simulink model "Kundur_BESS_STA_Nov14_2021a_v2_2021a"  (R2023a)
settings: Solver=VariableStepAuto  StartTime=0.0  StopTime=3  FixedStep=Ts  MaxStep=1e-5  MinStep=1e-20  RelTol=1e-3  EnableMultiTasking=on
PreLoadFcn:
  | Ts=50e-6;
PostLoadFcn:
  | Ts=50e-6;
InitFcn:
  | Ts=50e-6;
values from neighbouring files (symbols this model uses):
  current_K_den = [1 -1.95396088137 0.953960881373]    [param_cntrl_v2.mat]
  current_K_num = [292.549944556 -582.765243791 290.215658722]    [param_cntrl_v2.mat]
  flt_den = [1 -1.99914493247 0.999500180349]    [param_cntrl_v2.mat]
  flt_num = [0.000249925443627 3.12366678454e-08 -0.000249894206959]    [param_cntrl_v2.mat]
  flt_rocof_den = [1 -3.94812243331 5.84544117496 -3.84650440967 0.949185710471]    [param_cntrl_v2.mat]
  flt_rocof_num = [2.65341753303e-09 1.06136701321e-08 1.59205051982e-08 1.06136701321e-08 2.65341753303e-09]    [param_cntrl_v2.mat]
  pll_K_den = [1 -1.95396088137 0.953960881373]    [param_cntrl_v2.mat]
  pll_K_num = [1047.77474974 -2078.89023245 1031.12061217]    [param_cntrl_v2.mat]
  sampling_k = 5e-05    [param_cntrl_v2.mat]
undefined symbols (not defined in the file or in its folder): Ad2, Ad4, Bd2, Bd4, Cd2, Cd4, D1, Delta, flt_rocof_a_den, flt_rocof_a_num, flt_rocof_b_den, flt_rocof_b_num, Gd2, Gd4, Kd2, Kd4, L, R
libraries: spsThreePhaseVIMeasurementLib x15, spsLoadFlowBusLib x12, spsSeriesRLCBranchLib x11, spsThreePhaseSeriesRLCLoadLib x11, spsThreePhaseTransformerTwoWindingsLib x8, spsThreePhaseSeriesRLCBranchLib x8, spsabctoAlphaBetaZeroLib x8, spsGenericPowerSystemStabilizerLib x8, spsPowerPositiveSequenceLib x7, spsThreePhaseParallelRLCLoadLib x6, spsPLL3phLib x6, spsGroundLib x6
(part 3 of 4)

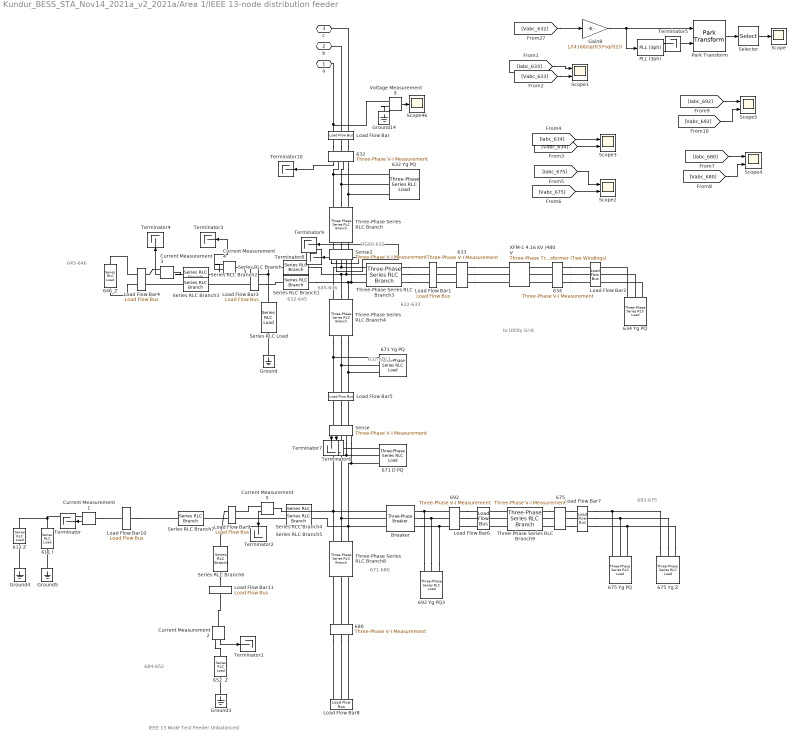
== system Kundur_BESS_STA_Nov14_2021a_v2_2021a/Area 1/IEEE 13-node distribution feeder ==
  note: 632-633
  note: 645-646
  note: 684-652
  note: 692-675
  note: 671-680
  note: 632-nDL1
  note: IEEE 13 Node Test Feeder Unbalanced
  note: 632-645
  note: RG60-632
  note: to Utility Grid
  note: 645-646
  " 634 Yg PQ " : spsThreePhaseSeriesRLCLoadLib/Three-Phase Series RLC Load  LConnTagsString=A|B|C  Configuration=Y (grounded)  NominalVoltage=120e3  Vabc=[ 1 1 1]*277.128  Vabcp=[1e3 1e3 1e3]  NominalFrequency=60  UnbalancedPower=on  ActivePower=1e+006  InductivePower=0  CapacitivePower=0  Pabc=[160 120 120]*1e3  QLabc=[110 90 90]*1e3  QCabc=[0 0 0]  Pabcp=[10e3 9e3 11e3]  QLabcp=[100 90 110]  QCabcp=[100 90 110]  Measurements=None  LoadType=constant PQ
      settings: AttributesFormatString=|
      | P= %<Pabc> W
      | Ql=%<QLabc> var
      | Qc=%<QCabc> var
  611 I : spsSeriesRLCLoadLib/Series RLC Load  LConnTagsString=a  RConnTagsString=__new0  NominalVoltage=0.986941*2401.78  NominalFrequency=60  ActivePower=50e3  InductivePower=80e3  CapacitivePower=0  Setx0=off  InitialVoltage=0  SetiL0=off  InitialCurrent=0  Measurements=None  LoadType=constant I
      settings: AttributesFormatString=|
      | P=%<ActivePower> W
      | Ql=%<InductivePower> var
      | Qc=%<CapacitivePower> var
  611 Z : spsSeriesRLCLoadLib/Series RLC Load  LConnTagsString=a  RConnTagsString=__new0  NominalVoltage=4160/sqrt(3)  NominalFrequency=60  ActivePower=0  InductivePower=0  CapacitivePower=100e3  Setx0=off  InitialVoltage=0  SetiL0=off  InitialCurrent=0  Measurements=None  LoadType=constant Z
      settings: AttributesFormatString=|
      | P=%<ActivePower> W
      | Ql=%<InductivePower> var
      | Qc=%<CapacitivePower> var
  632 : spsThreePhaseVIMeasurementLib/Three-Phase V-I Measurement  VoltageMeasurement=phase-to-ground  SetLabelV=on  LabelV=Vabc_632  Vpu=off  VpuLL=off  CurrentMeasurement=yes  SetLabelI=off  LabelI=Iabc_632  Ipu=off  Pbase=100e6  Vbase=4160  OutputType=Complex  PhasorSimulation=off  PSBequivalent=0
  632 Yg PQ : spsThreePhaseSeriesRLCLoadLib/Three-Phase Series RLC Load  LConnTagsString=A|B|C  Configuration=Y (grounded)  NominalVoltage=120e3  Vabc=[ 1.021 1.042 1.0174]*2401.78  Vabcp=[1e3 1e3 1e3]  NominalFrequency=60  UnbalancedPower=on  ActivePower=1e+006  InductivePower=0  CapacitivePower=0  Pabc="[17 66  117]*1e3/2"  QLabc="[10 38  68]*1e3/2"  QCabc=[0 0 0]  Pabcp=[10e3 9e3 11e3]  QLabcp=[100 90 110]  QCabcp=[100 90 110]  Measurements=None  LoadType=constant PQ
      settings: AttributesFormatString=|
      | P= %<Pabc> W
      | Ql=%<QLabc> var
      | Qc=%<QCabc> var
  633 : spsThreePhaseVIMeasurementLib/Three-Phase V-I Measurement  VoltageMeasurement=phase-to-ground  SetLabelV=on  LabelV=Vabc_633  Vpu=off  VpuLL=off  CurrentMeasurement=yes  SetLabelI=on  LabelI=Iabc_633  Ipu=off  Pbase=100e6  Vbase=4160  OutputType=Complex  PhasorSimulation=off  PSBequivalent=0
  634 : spsThreePhaseVIMeasurementLib/Three-Phase V-I Measurement  VoltageMeasurement=phase-to-ground  SetLabelV=on  LabelV=Vabc_634  Vpu=off  VpuLL=off  CurrentMeasurement=yes  SetLabelI=on  LabelI=Iabc_634  Ipu=off  Pbase=100e6  Vbase=4160  OutputType=Complex  PhasorSimulation=off  PSBequivalent=0
  646_Z : spsSeriesRLCLoadLib/Series RLC Load  LConnTagsString=a  RConnTagsString=__new0  NominalVoltage=4160  NominalFrequency=60  ActivePower=30e3  InductivePower=132e3  CapacitivePower=0  Setx0=off  InitialVoltage=0  SetiL0=off  InitialCurrent=0  Measurements=None  LoadType=constant Z
      settings: AttributesFormatString=|
      | P=%<ActivePower> W
      | Ql=%<InductivePower> var
      | Qc=%<CapacitivePower> var
  "652  Z " : spsSeriesRLCLoadLib/Series RLC Load  LConnTagsString=a  RConnTagsString=__new0  NominalVoltage=4160/sqrt(3)  NominalFrequency=60  ActivePower=128e3*0.1  InductivePower=86e3  CapacitivePower=0  Setx0=off  InitialVoltage=0  SetiL0=off  InitialCurrent=0  Measurements=None  LoadType=constant Z
      settings: AttributesFormatString=|
      | P=%<ActivePower> W
      | Ql=%<InductivePower> var
      | Qc=%<CapacitivePower> var
  671 D PQ : spsThreePhaseSeriesRLCLoadLib/Three-Phase Series RLC Load  LConnTagsString=A|B|C  Configuration=Delta  NominalVoltage=120e3  Vabc="[1  1  1]*120e3/sqrt(3)"  Vabcp=[ 1.73773 1.77224 1.71484]*2401.78  NominalFrequency=60  UnbalancedPower=on  ActivePower=1e+006  InductivePower=0  CapacitivePower=0  Pabc="[17 66  117]*1e3/2"  QLabc="[10 38  68]*1e3/2"  QCabc=[0 0 0]  Pabcp=[385 385 385 ]*1e3  QLabcp=[220 220 220]*1e3  QCabcp="[0  0  0]"  Measurements=None  LoadType=constant PQ
      settings: AttributesFormatString=|
      | P= %<Pabcp> W
      | Ql=%<QLabcp> var
      | Qc=%<QCabcp> var
  671 Yg PQ : spsThreePhaseSeriesRLCLoadLib/Three-Phase Series RLC Load  LConnTagsString=A|B|C  Configuration=Y (grounded)  NominalVoltage=120e3  Vabc=[ 0.987076 1.0519 0.978043]*2401.78  Vabcp=[1e3 1e3 1e3]  NominalFrequency=60  UnbalancedPower=on  ActivePower=1e+006  InductivePower=0  CapacitivePower=0  Pabc="[17 66  117]*1e3/2"  QLabc="[10 38  68]*1e3/2"  QCabc=[0 0 0]  Pabcp=[10e3 9e3 11e3]  QLabcp=[100 90 110]  QCabcp=[100 90 110]  Measurements=None  LoadType=constant PQ
      settings: AttributesFormatString=|
      | P= %<Pabc> W
      | Ql=%<QLabc> var
      | Qc=%<QCabc> var
  675 : spsThreePhaseVIMeasurementLib/Three-Phase V-I Measurement  VoltageMeasurement=phase-to-ground  SetLabelV=on  LabelV=Vabc_675  Vpu=off  VpuLL=off  CurrentMeasurement=yes  SetLabelI=on  LabelI=Iabc_675  Ipu=off  Pbase=100e6  Vbase=4160  OutputType=Complex  PhasorSimulation=off  PSBequivalent=0
  675 Yg PQ : spsThreePhaseSeriesRLCLoadLib/Three-Phase Series RLC Load  LConnTagsString=A|B|C  Configuration=Y (grounded)  NominalVoltage=120e3  Vabc=[ 0.98063 1.05431 0.975983]*2401.78  Vabcp=[1e3 1e3 1e3]  NominalFrequency=60  UnbalancedPower=on  ActivePower=1e+006  InductivePower=0  CapacitivePower=0  Pabc="[485  68  290]*1e3"  QLabc="[190  60  212]*1e3"  QCabc=[0 0 0]  Pabcp=[10e3 9e3 11e3]  QLabcp=[100 90 110]  QCabcp=[100 90 110]  Measurements=None  LoadType=constant PQ
      settings: AttributesFormatString=|
      | P= %<Pabc> W
      | Ql=%<QLabc> var
      | Qc=%<QCabc> var
  675 Yg Z : spsThreePhaseSeriesRLCLoadLib/Three-Phase Series RLC Load  LConnTagsString=A|B|C  Configuration=Y (grounded)  NominalVoltage=120e3  Vabc=[ 1 1 1]*2401.78  Vabcp=[1e3 1e3 1e3]  NominalFrequency=60  UnbalancedPower=on  ActivePower=1e+006  InductivePower=0  CapacitivePower=0  Pabc=[0 0 0]  QLabc=[0 0 0]  QCabc=[200 200 200]*1e3  Pabcp=[10e3 9e3 11e3]  QLabcp=[100 90 110]  QCabcp=[100 90 110]  Measurements=None  LoadType=constant Z
      settings: AttributesFormatString=|
      | P= %<Pabc> W
      | Ql=%<QLabc> var
      | Qc=%<QCabc> var
  680 : spsThreePhaseVIMeasurementLib/Three-Phase V-I Measurement  VoltageMeasurement=phase-to-ground  SetLabelV=on  LabelV=Vabc_680  Vpu=off  VpuLL=off  CurrentMeasurement=yes  SetLabelI=on  LabelI=Iabc_680  Ipu=off  Pbase=100e6  Vbase=4160  OutputType=Complex  PhasorSimulation=off  PSBequivalent=0
  692 : spsThreePhaseVIMeasurementLib/Three-Phase V-I Measurement  VoltageMeasurement=phase-to-ground  SetLabelV=on  LabelV=Vabc_692  Vpu=off  VpuLL=off  CurrentMeasurement=yes  SetLabelI=on  LabelI=Iabc_692  Ipu=off  Pbase=100e6  Vbase=4160  OutputType=Complex  PhasorSimulation=off  PSBequivalent=0
  692 Yg PQ3 : spsThreePhaseSeriesRLCLoadLib/Three-Phase Series RLC Load  LConnTagsString=A|B|C  Configuration=Y (grounded)  NominalVoltage=120e3  Vabc=[ 1.73488 1.75203 1.72341]*2401.78  Vabcp=[1e3 1e3 1e3]  NominalFrequency=60  UnbalancedPower=on  ActivePower=1e+006  InductivePower=0  CapacitivePower=0  Pabc=[1e-6 1e-6 170 ]*1e3  QLabc=[3000 3000 3000]*1e3  QCabc=[0 0 0]  Pabcp=[10e3 9e3 11e3]  QLabcp=[100 90 110]  QCabcp=[100 90 110]  Measurements=None  LoadType=constant PQ
      settings: AttributesFormatString=|
      | P= %<Pabc> W
      | Ql=%<QLabc> var
      | Qc=%<QCabc> var
  Breaker : spsThreePhaseBreakerLib/Three-Phase Breaker  InitialState=closed  SwitchA=on  SwitchB=on  SwitchC=on  SwitchTimes=[0]  External=off  BreakerResistance=0.001  SnubberResistance=1e3  SnubberCapacitance=1e-4  Measurements=None
  Current Measurement{1..5} (5 alike) : spsCurrentMeasurementLib/Current Measurement  PhasorSimulation=off  OutputType=Complex  PSBequivalent=0
  Gain8 : Gain  Gain=1/(4160/sqrt(3)*sqrt(2))
  Ground{,3..5,14} (5 alike) : spsGroundLib/Ground  LConnTagsString=a
  Load Flow Bar : spsLoadFlowBusLib/Load Flow Bus  LConnTagsString=a|b|c  RConnTagsString=a|b|c  Phases=ABC  Connectors=on both sides  ID=632  Vbase=2401.78  Vref="[ 1  1  1]"  Vangle="[ 0  -120  120]"  VLF=1.021  VLFb=1.042  VLFc=1.017  angleLF=-2.49  angleLFb=-121.7  angleLFc=117.8
      settings: AttributesFormatString=%<ID>
  Load Flow Bar1 : spsLoadFlowBusLib/Load Flow Bus  LConnTagsString=a|b|c  RConnTagsString=a|b|c  Phases=ABC  Connectors=on both sides  ID=633  Vbase=2401.78  Vref=[1.0 1.0 1.0]  Vangle=[0 -120 120]  VLF=0.9671  VLFb=0.9801  VLFc=0.9575  angleLF=-5.793  angleLFb=-125.9  angleLFc=113.9
      settings: AttributesFormatString=%<ID>
  Load Flow Bar10 : spsLoadFlowBusLib/Load Flow Bus  LConnTagsString=a  RConnTagsString=a  Phases=C  Connectors=on both sides  ID=611  Vbase=2401.78  Vref=[1.0 1.0 1.0]  Vangle=[0 -120 120]  VLF=NaN  VLFb=NaN  VLFc=0.9623  angleLF=NaN  angleLFb=NaN  angleLFc=112.9
      settings: AttributesFormatString=%<ID>
  Load Flow Bar11 : spsLoadFlowBusLib/Load Flow Bus  LConnTagsString=a  RConnTagsString=a  Phases=A  Connectors=on both sides  ID=652  Vbase=2401.78  Vref=[1.0 1.0 1.0]  Vangle=[0 -120 120]  VLF=0.969  VLFb=NaN  VLFc=NaN  angleLF=-6.548  angleLFb=NaN  angleLFc=NaN
      settings: AttributesFormatString=%<ID>
  Load Flow Bar2 : spsLoadFlowBusLib/Load Flow Bus  LConnTagsString=a|b|c  RConnTagsString=a|b|c  Phases=ABC  Connectors=on both sides  ID=634  Vbase=480/sqrt(3)  Vref="[1  1  1 ]"  Vangle=[0 -120 120]  VLF=0.9473  VLFb=0.9605  VLFc=0.9374  angleLF=-6.323  angleLFb=-126.4  angleLFc=113.4
      settings: AttributesFormatString=%<ID>
  Load Flow Bar3 : spsLoadFlowBusLib/Load Flow Bus  LConnTagsString=a|b  RConnTagsString=a|b  Phases=BC  Connectors=on both sides  ID=645  Vbase=2401.78  Vref=[1 1 1]  Vangle=[0 -120 120]  VLF=NaN  VLFb=0.982  VLFc=0.9645  angleLF=NaN  angleLFb=-126.4  angleLFc=113.8
      settings: AttributesFormatString=%<ID>
  Load Flow Bar4 : spsLoadFlowBusLib/Load Flow Bus  LConnTagsString=a|b  RConnTagsString=a|b  Phases=BC  Connectors=on both sides  ID=646  Vbase=2401.78  Vref=[1 1 1]  Vangle=[0 -120 120]  VLF=NaN  VLFb=0.9803  VLFc=0.9619  angleLF=NaN  angleLFb=-126.5  angleLFc=113.8
      settings: AttributesFormatString=%<ID>
  Load Flow Bar5 : spsLoadFlowBusLib/Load Flow Bus  LConnTagsString=a|b|c  RConnTagsString=a|b|c  Phases=ABC  Connectors=on both sides  ID=671  Vbase=2401.78  Vref=[1.0 1.0 1.0]  Vangle=[0 -120 120]  VLF=0.9734  VLFb=0.988  VLFc=0.9653  angleLF=-6.515  angleLFb=-126.5  angleLFc=113.1
      settings: AttributesFormatString=%<ID>
  Load Flow Bar6 : spsLoadFlowBusLib/Load Flow Bus  LConnTagsString=a|b|c  RConnTagsString=a|b|c  Phases=ABC  Connectors=on both sides  ID=692  Vbase=2401.78  Vref=[1 1 1]  Vangle=[0 -120 120]  VLF=0.9734  VLFb=0.988  VLFc=0.9653  angleLF=-6.515  angleLFb=-126.5  angleLFc=113.1
      settings: AttributesFormatString=%<ID>
  Load Flow Bar7 : spsLoadFlowBusLib/Load Flow Bus  LConnTagsString=a|b|c  RConnTagsString=a|b|c  Phases=ABC  Connectors=on both sides  ID=675  Vbase=2401.78  Vref=[1 1 1]  Vangle=[0 -120 120]  VLF=0.9761  VLFb=0.9908  VLFc=0.9679  angleLF=-6.673  angleLFb=-126.7  angleLFc=113
      settings: AttributesFormatString=%<ID>
  Load Flow Bar8 : spsLoadFlowBusLib/Load Flow Bus  LConnTagsString=a|b|c  Phases=ABC  Connectors=on one side  ID=680  Vbase=2401.78  Vref=[1 1 1]  Vangle=[0 -120 120]  VLF=0.9734  VLFb=0.988  VLFc=0.9653  angleLF=-6.515  angleLFb=-126.5  angleLFc=113.1
      settings: AttributesFormatString=%<ID>
  Load Flow Bar9 : spsLoadFlowBusLib/Load Flow Bus  LConnTagsString=a|b  RConnTagsString=a|b  Phases=AC  Connectors=on both sides  ID=684  Vbase=2401.78  Vref=[1.0 1.0 1.0]  Vangle=[0 -120 120]  VLF=0.9709  VLFb=NaN  VLFc=0.9635  angleLF=-6.557  angleLFb=NaN  angleLFc=113
      settings: AttributesFormatString=%<ID>
  PLL (3ph) : spsPLL3phLib/PLL (3ph)  Fmin=45  Par_Init=[0, 60]  ParK=[180, 3200, 1]  TcD=1e-4  MaxRateChangeFreq=12  FilterCutOffFreq=25  Ts=0  AGC=on
  Park Transform : eeTransforms/Park Transform  AxisAlignment=Q-axis  PowerInvariant=off
  Scope : Scope
  Scope{1..5} (5 alike) : Scope  NumInputPorts=2
  Scope46 : Scope
  Selector : Selector  InputPortWidth=3  IndexOptions=Index vector (dialog)  Indices=[1]  OutputSizes=1
  Sense : spsThreePhaseVIMeasurementLib/Three-Phase V-I Measurement  VoltageMeasurement=phase-to-ground  SetLabelV=off  LabelV=Vabc_sense  Vpu=off  VpuLL=off  CurrentMeasurement=yes  SetLabelI=off  LabelI=Iabc_sense  Ipu=off  Pbase=100e6  Vbase=4160  OutputType=Complex  PhasorSimulation=off  PSBequivalent=0
  Sense2 : spsThreePhaseVIMeasurementLib/Three-Phase V-I Measurement  VoltageMeasurement=phase-to-ground  SetLabelV=off  LabelV=Vabc_sense2  Vpu=off  VpuLL=off  CurrentMeasurement=yes  SetLabelI=off  LabelI=Iabc_sense2  Ipu=off  Pbase=100e6  Vbase=4160  OutputType=Complex  PhasorSimulation=off  PSBequivalent=0
  Series RLC Branch : spsSeriesRLCBranchLib/Series RLC Branch  LConnTagsString=__new0  RConnTagsString=__new0  BranchType=RLC  Resistance=R.line5  Inductance=L.line5  SetiL0=off  InitialCurrent=0  Capacitance=0  Setx0=off  InitialVoltage=0  Measurements=None
  Series RLC Branch1 : spsSeriesRLCBranchLib/Series RLC Branch  LConnTagsString=__new0  RConnTagsString=__new0  BranchType=RLC  Resistance=R.line5  Inductance=L.line5  SetiL0=off  InitialCurrent=0  Capacitance=0  Setx0=off  InitialVoltage=0  Measurements=None
  Series RLC Branch2 : spsSeriesRLCBranchLib/Series RLC Branch  LConnTagsString=__new0  RConnTagsString=__new0  BranchType=RLC  Resistance=R.line2  Inductance=L.line2  SetiL0=off  InitialCurrent=0  Capacitance=0  Setx0=off  InitialVoltage=0  Measurements=None
  Series RLC Branch3 : spsSeriesRLCBranchLib/Series RLC Branch  LConnTagsString=__new0  RConnTagsString=__new0  BranchType=RLC  Resistance=R.line2  Inductance=L.line2  SetiL0=off  InitialCurrent=0  Capacitance=0  Setx0=off  InitialVoltage=0  Measurements=None
  Series RLC Branch4 : spsSeriesRLCBranchLib/Series RLC Branch  LConnTagsString=__new0  RConnTagsString=__new0  BranchType=RLC  Resistance=R.line7  Inductance=L.line7  SetiL0=off  InitialCurrent=0  Capacitance=0  Setx0=off  InitialVoltage=0  Measurements=None
  Series RLC Branch5 : spsSeriesRLCBranchLib/Series RLC Branch  LConnTagsString=__new0  RConnTagsString=__new0  BranchType=RLC  Resistance=R.line7  Inductance=L.line7  SetiL0=off  InitialCurrent=0  Capacitance=0  Setx0=off  InitialVoltage=0  Measurements=None
  Series RLC Branch6 : spsSeriesRLCBranchLib/Series RLC Branch  LConnTagsString=__new0  RConnTagsString=__new0  BranchType=RLC  Resistance=R.line8  Inductance=L.line8  SetiL0=off  InitialCurrent=0  Capacitance=0  Setx0=off  InitialVoltage=0  Measurements=None
  Series RLC Branch7 : spsSeriesRLCBranchLib/Series RLC Branch  LConnTagsString=__new0  RConnTagsString=__new0  BranchType=RLC  Resistance=R.line7  Inductance=L.line7  SetiL0=off  InitialCurrent=0  Capacitance=0  Setx0=off  InitialVoltage=0  Measurements=None
  Series RLC Load : spsSeriesRLCLoadLib/Series RLC Load  LConnTagsString=a  RConnTagsString=__new0  NominalVoltage=2401.78  NominalFrequency=60  ActivePower=70e3  InductivePower=125e3  CapacitivePower=0  Setx0=off  InitialVoltage=0  SetiL0=off  InitialCurrent=0  Measurements=None  LoadType=constant Z
  Terminator{,1..10} (11 alike) : Terminator
  Three-Phase Series RLC Branch : spsThreePhaseSeriesRLCBranchLib/Three-Phase Series RLC Branch  LConnTagsString=A|B|C  RConnTagsString=A|B|C  BranchType=RLC  Resistance=R.line1  Inductance=L.line1  Capacitance=0  Measurements=None
  Three-Phase Series RLC Branch3 : spsThreePhaseSeriesRLCBranchLib/Three-Phase Series RLC Branch  LConnTagsString=A|B|C  RConnTagsString=A|B|C  BranchType=RLC  Resistance=R.line3  Inductance=L.line3  Capacitance=0  Measurements=None
  Three-Phase Series RLC Branch4 : spsThreePhaseSeriesRLCBranchLib/Three-Phase Series RLC Branch  LConnTagsString=A|B|C  RConnTagsString=A|B|C  BranchType=RLC  Resistance=R.line4  Inductance=L.line4  Capacitance=0  Measurements=None
  Three-Phase Series RLC Branch8 : spsThreePhaseSeriesRLCBranchLib/Three-Phase Series RLC Branch  LConnTagsString=A|B|C  RConnTagsString=A|B|C  BranchType=RLC  Resistance=R.line10  Inductance=L.line10  Capacitance=0  Measurements=None
  Three-Phase Series RLC Branch9 : spsThreePhaseSeriesRLCBranchLib/Three-Phase Series RLC Branch  LConnTagsString=A|B|C  RConnTagsString=A|B|C  BranchType=RLC  Resistance=R.line11  Inductance=L.line11  Capacitance=0  Measurements=None
  Voltage Measurement9 : spsVoltageMeasurementLib/Voltage Measurement  PhasorSimulation=off  OutputType=Complex  PSBequivalent=0
  XFM-1 4.16 kV /480 V : spsThreePhaseTransformerTwoWindingsLib/Three-Phase Transformer (Two Windings)  Winding1Connection=Yg  Winding2Connection=Yg  CoreType=Three single-phase transformers  SetSaturation=off  Hysteresis=off  DataFile='hysteresis'  SetInitialFlux=off  Measurements=None  UNITS=pu  NominalPower=[ 500e3 , 60 ]  Winding1=[4160 0.011 0.02]  Winding2=[480 0 0]  Rm=500  Lm=500  L0=0.5  Saturation=[0 0;0.0024 1.2;1 1.52]  InitialFluxes=[0.8 -0.8 0.7]  BreakLoop=off  DiscreteSolver=Trapezoidal iterative  DataType=off  TransfoNumber=1
  a : PMIOPort  Side=Left
  b : PMIOPort  Port=2  Side=Left
  c : PMIOPort  Port=3  Side=Left
  wires:
  Voltage Measurement9/1 -> Scope46/1
  PLL (3ph)/2 -> Park Transform/2
  [Vabc_632] -> Gain8/1
  Park Transform/1 -> Selector/1
  Gain8/1 -> PLL (3ph)/1, Park Transform/1
  Selector/1 -> Scope/1
  Current Measurement1/1 -> Terminator/1
  Current Measurement2/1 -> Terminator1/1
  Current Measurement5/1 -> Terminator2/1
  Current Measurement4/1 -> Terminator3/1
  Current Measurement3/1 -> Terminator4/1
  [Iabc_633] -> Scope1/1
  PLL (3ph)/1 -> Terminator5/1
  [Vabc_633] -> Scope1/2
  [Iabc_634] -> Scope3/1
  [Vabc_634] -> Scope3/2
  [Iabc_675] -> Scope2/1
  [Vabc_675] -> Scope2/2
  [Vabc_680] -> Scope4/2
  [Iabc_680] -> Scope4/1
  [Iabc_692] -> Scope5/1
  [Vabc_692] -> Scope5/2
  Sense/2 -> Terminator6/1
  Sense/1 -> Terminator7/1
  Sense2/1 -> Terminator8/1
  Sense2/2 -> Terminator9/1
  632/1 -> Terminator10/1
  connections:
  Sense/LConn2 -- Load Flow Bar5/RConn2
  680/LConn2 -- Three-Phase Series RLC Branch8/LConn2
  692 Yg PQ3/LConn2 -- Breaker/RConn2 -- 692/LConn2
  680/RConn3 -- Load Flow Bar8/LConn3
  Three-Phase Series RLC Branch8/RConn2 -- Sense/RConn2 -- 671 D PQ/LConn2 -- Breaker/LConn2
  675 Yg Z/LConn1 -- 675 Yg PQ/LConn1 -- Load Flow Bar7/LConn1
  675/LConn2 -- Three-Phase Series RLC Branch9/RConn2
  Current Measurement3/RConn1 -- Load Flow Bar4/RConn1
  Load Flow Bar3/RConn2 -- Series RLC Branch1/LConn1
  Three-Phase Series RLC Branch/RConn2 -- 632 Yg PQ/LConn2 -- 632/RConn2
  Current Measurement5/RConn1 -- Load Flow Bar9/RConn1
  Three-Phase Series RLC Branch3/LConn2 -- Load Flow Bar1/LConn2
  Sense2/RConn1 -- Three-Phase Series RLC Branch4/RConn1 -- Three-Phase Series RLC Branch3/RConn1
  680/RConn1 -- Load Flow Bar8/LConn1
  Current Measurement3/LConn1 -- Series RLC Branch2/LConn1
  Series RLC Branch6/LConn1 -- Load Flow Bar9/LConn1
  Three-Phase Series RLC Branch3/LConn1 -- Load Flow Bar1/LConn1
  Three-Phase Series RLC Branch3/LConn3 -- Load Flow Bar1/LConn3
  634/LConn3 -- XFM-1 4.16 kV /480 V/RConn3
  " 634 Yg PQ "/LConn3 -- Load Flow Bar2/RConn3
  Three-Phase Series RLC Branch9/LConn3 -- Load Flow Bar6/LConn3
  Voltage Measurement9/LConn2 -- Ground14/LConn1
  680/LConn1 -- Three-Phase Series RLC Branch8/LConn1
  634/LConn2 -- XFM-1 4.16 kV /480 V/RConn2
  675 Yg Z/LConn2 -- 675 Yg PQ/LConn2 -- Load Flow Bar7/LConn2
  Sense2/RConn2 -- Series RLC Branch/RConn1 -- Three-Phase Series RLC Branch4/RConn2 -- Three-Phase Series RLC Branch3/RConn2
  Current Measurement2/LConn1 -- Load Flow Bar11/RConn1
  Three-Phase Series RLC Branch9/LConn2 -- Load Flow Bar6/LConn2
  Sense2/LConn1 -- Three-Phase Series RLC Branch/LConn1
  692/RConn1 -- Load Flow Bar6/RConn1
  Three-Phase Series RLC Branch4/LConn2 -- 671 Yg PQ/LConn2 -- Load Flow Bar5/LConn2
  Sense/LConn3 -- Load Flow Bar5/RConn3
  Series RLC Branch3/LConn1 -- Load Flow Bar4/RConn2
  Three-Phase Series RLC Branch/RConn1 -- 632 Yg PQ/LConn1 -- 632/RConn1
  Current Measurement4/LConn1 -- Load Flow Bar3/LConn1
  692 Yg PQ3/LConn3 -- Breaker/RConn3 -- 692/LConn3
  Series RLC Load/LConn1 -- Series RLC Branch/LConn1 -- Load Flow Bar3/RConn1
  675 Yg Z/LConn3 -- 675 Yg PQ/LConn3 -- Load Flow Bar7/LConn3
  633/RConn1 -- XFM-1 4.16 kV /480 V/LConn1
  680/RConn2 -- Load Flow Bar8/LConn2
  671 Yg PQ/LConn1 -- Three-Phase Series RLC Branch4/LConn1 -- Load Flow Bar5/LConn1
  Three-Phase Series RLC Branch/RConn3 -- 632 Yg PQ/LConn3 -- 632/RConn3
  Current Measurement4/RConn1 -- Series RLC Branch2/RConn1
  Load Flow Bar10/RConn1 -- Series RLC Branch7/LConn1
  Three-Phase Series RLC Branch4/RConn3 -- Sense2/RConn3 -- Three-Phase Series RLC Branch3/RConn3 -- Series RLC Branch1/RConn1
  " 634 Yg PQ "/LConn2 -- Load Flow Bar2/RConn2
  692/RConn3 -- Load Flow Bar6/RConn3
  Voltage Measurement9/LConn1 -- Load Flow Bar/LConn1 -- a/RConn1
  675/LConn1 -- Three-Phase Series RLC Branch9/RConn1
  680/LConn3 -- Three-Phase Series RLC Branch8/LConn3
  Three-Phase Series RLC Branch4/LConn3 -- Load Flow Bar5/LConn3 -- 671 Yg PQ/LConn3
  Sense/LConn1 -- Load Flow Bar5/RConn1
  Load Flow Bar3/LConn2 -- Series RLC Branch3/RConn1
  633/LConn2 -- Load Flow Bar1/RConn2
  Ground5/LConn1 -- 611 I/RConn1
  675/RConn3 -- Load Flow Bar7/RConn3
  692/RConn2 -- Load Flow Bar6/RConn2
  633/LConn3 -- Load Flow Bar1/RConn3
  Load Flow Bar/RConn1 -- 632/LConn1
  Series RLC Branch6/RConn1 -- Load Flow Bar11/LConn1
  " 634 Yg PQ "/LConn1 -- Load Flow Bar2/RConn1
  Current Measurement1/LConn1 -- Load Flow Bar10/LConn1
  675/LConn3 -- Three-Phase Series RLC Branch9/RConn3
  633/LConn1 -- Load Flow Bar1/RConn1
  Load Flow Bar4/LConn2 -- 646_Z/RConn1
  Load Flow Bar/RConn3 -- 632/LConn3
  Ground/LConn1 -- Series RLC Load/RConn1
  Load Flow Bar/RConn2 -- 632/LConn2
  634/LConn1 -- XFM-1 4.16 kV /480 V/RConn1
  Current Measurement5/LConn1 -- Series RLC Branch4/LConn1
  633/RConn2 -- XFM-1 4.16 kV /480 V/LConn2
  Breaker/LConn1 -- Series RLC Branch4/RConn1 -- Sense/RConn1 -- 671 D PQ/LConn1 -- Three-Phase Series RLC Branch8/RConn1
  Breaker/LConn3 -- Series RLC Branch5/RConn1 -- Sense/RConn3 -- 671 D PQ/LConn3 -- Three-Phase Series RLC Branch8/RConn3
  Current Measurement2/RConn1 -- "652  Z "/LConn1
  Ground3/LConn1 -- "652  Z "/RConn1
  692 Yg PQ3/LConn1 -- Breaker/RConn1 -- 692/LConn1
  634/RConn1 -- Load Flow Bar2/LConn1
  634/RConn2 -- Load Flow Bar2/LConn2
  Ground4/LConn1 -- 611 Z/RConn1
  Sense2/LConn3 -- Three-Phase Series RLC Branch/LConn3
  Load Flow Bar9/LConn2 -- Series RLC Branch7/RConn1
  Series RLC Branch5/LConn1 -- Load Flow Bar9/RConn2
  675/RConn2 -- Load Flow Bar7/RConn2
  Sense2/LConn2 -- Three-Phase Series RLC Branch/LConn2
  Three-Phase Series RLC Branch9/LConn1 -- Load Flow Bar6/LConn1
  634/RConn3 -- Load Flow Bar2/LConn3
  Load Flow Bar4/LConn1 -- 646_Z/LConn1
  675/RConn1 -- Load Flow Bar7/RConn1
  633/RConn3 -- XFM-1 4.16 kV /480 V/LConn3
  Current Measurement1/RConn1 -- 611 Z/LConn1 -- 611 I/LConn1
  Load Flow Bar/LConn2 -- b/RConn1
  Load Flow Bar/LConn3 -- c/RConn1

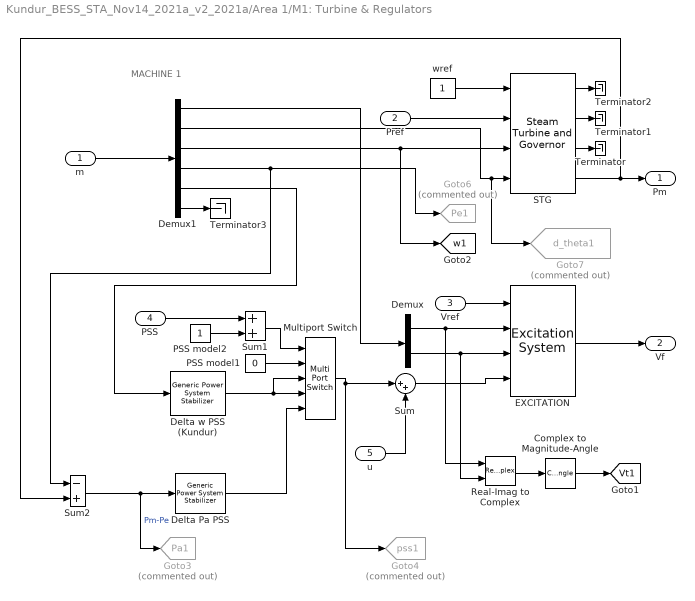
== system Kundur_BESS_STA_Nov14_2021a_v2_2021a/Area 1/M1: Turbine & Regulators ==
  note: MACHINE 1
  m : Inport
  Pref : Inport  Port=2
  Vref : Inport  Port=3
  PSS : Inport  Port=4
  u : Inport  Port=5
  Complex to Magnitude-Angle : ComplexToMagnitudeAngle  Output=Magnitude
  Delta Pa PSS : spsGenericPowerSystemStabilizerLib/Generic Power System Stabilizer  Tsensor=15e-3  K=2.5*1.25  Twashout=1  Tleadlag1=[60e-3 1]  Tleadlag2=[0 0]  VSlimits=[-0.15 0.15]  Vinit=0  Plot_On=off  MagdB_On=on  FreqRange=logspace(-2,2,500)
  Delta w PSS (Kundur) : spsGenericPowerSystemStabilizerLib/Generic Power System Stabilizer  Tsensor=15e-3  K=30  Twashout=10  Tleadlag1=[50e-3 20e-3]  Tleadlag2=[3 5.4]  VSlimits=[-0.15 0.15]  Vinit=0  Plot_On=off  MagdB_On=on  FreqRange=logspace(-2,2,500)
  Demux : Demux  Outputs=2
      settings: DisplayOption=none
  Demux1 : Demux  Outputs=[2 1 1 1 1 1]
  EXCITATION : spsExcitationSystemLib/Excitation System  tr=20e-3  reg=[ 200, 0.001 ]  exc=[ 1, 0 ]  tgr=[ 0, 0 ]  damp=[ 0, 0 ]  sat=[ 0, 0 ]  lim=[-12.3 , 12.3, 0 ]  v0=[1,1.83395]
  Goto3 : Goto  Commented=on  GotoTag=Pa1  TagVisibility=global
  Goto4 : Goto  Commented=on  GotoTag=pss1  TagVisibility=global
  Goto6 : Goto  Commented=on  GotoTag=Pe1  TagVisibility=global
  Goto7 : Goto  Commented=on  GotoTag=d_theta1  TagVisibility=global
  Multiport Switch : MultiPortSwitch  Inputs=4  SaturateOnIntegerOverflow=off
  PSS model1 : Constant  Value=0
  PSS model2 : Constant
  Real-Imag to Complex : RealImagToComplex
  STG : spsSteamTurbineandGovernorLib/Steam Turbine and Governor  gentype=Tandem-compound (single mass)  reg1="[ 1  0.05    0 ]"  reg2="[ 0.001  0.15 ]"  reg3="[ -0.1  0.1  0  4.496 ]"  N=3600  turb1="[ 0  10   3.3   0.5   ]"  turb2="[   0   0.36    0.36   0.28   ]"  HA="[ 0.046  1.430  1.465   0.192 ]"  KA="[ 90.44  53.88  64.59   62.94  ]"  DA="[ 0.0115  0.3575  0.3663   0.0137  ]"  ini1=0.7778  ini2=[0.779316,-31.4247]
  Sum : Sum  Inputs=|++
  Sum1 : Sum  InputSameDT=on  SaturateOnIntegerOverflow=on  OutDataTypeStr=Inherit: Same as first input
  Sum2 : Sum  Inputs=-+  InputSameDT=on  SaturateOnIntegerOverflow=on  OutDataTypeStr=Inherit: Same as first input
  Terminator{,1..3} (4 alike) : Terminator
  wref : Constant
  Pm : Outport  InitialOutput=0  VectorParamsAs1DForOutWhenUnconnected=off
  Vf : Outport  Port=2  InitialOutput=0  VectorParamsAs1DForOutWhenUnconnected=off
  tag scope: Vt1=global, w1=global
  wires:
  Demux/1 -> Real-Imag to Complex/1, EXCITATION/2
  Demux/2 -> Real-Imag to Complex/2, EXCITATION/3
  wref/1 -> STG/1
  Pref/1 -> STG/2
  m/1 -> Demux1/1
  Vref/1 -> EXCITATION/1
  Real-Imag to Complex/1 -> Complex to Magnitude-Angle/1
  EXCITATION/1 -> Vf/1
  Complex to Magnitude-Angle/1 -> [Vt1]
  Demux1/6 -> Terminator3/1
  PSS model1/1 -> Multiport Switch/2
  Delta w PSS (Kundur)/1 -> Multiport Switch/4, Multiport Switch/3
  Delta Pa PSS/1 -> Multiport Switch/5
  PSS model2/1 -> Sum1/2
  Sum1/1 -> Multiport Switch/1
  PSS/1 -> Sum1/1
  Demux1/1 -> Demux/1
  Demux1/3 -> [w1], STG/3
  Demux1/4 -> Sum2/1, Goto6/1
  Demux1/5 -> Delta w PSS (Kundur)/1
  Sum2/1 -> Delta Pa PSS/1, Goto3/1  "Pm-Pe"
  STG/3 -> Terminator/1
  Demux1/2 -> Goto7/1, STG/4
  STG/4 -> Pm/1, Sum2/2
  STG/2 -> Terminator1/1
  STG/1 -> Terminator2/1
  Multiport Switch/1 -> Sum/1, Goto4/1
  Sum/1 -> EXCITATION/4
  u/1 -> Sum/2

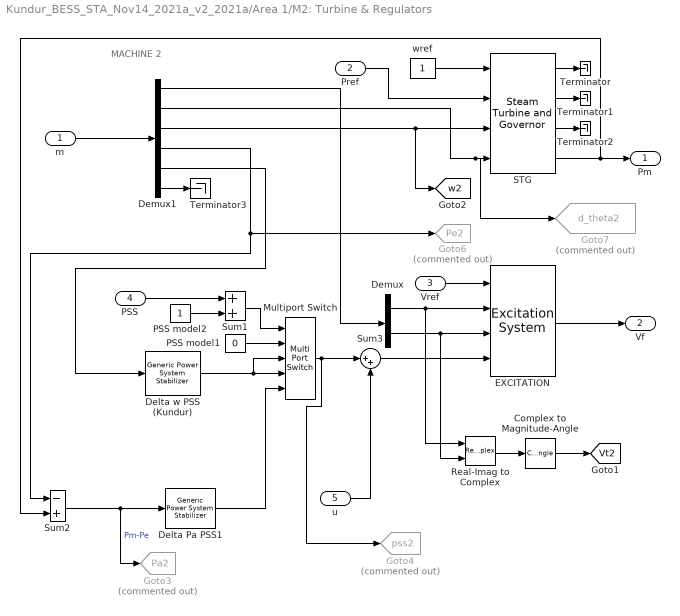
== system Kundur_BESS_STA_Nov14_2021a_v2_2021a/Area 1/M2: Turbine & Regulators ==
  note: MACHINE 2
  m : Inport
  Pref : Inport  Port=2
  Vref : Inport  Port=3
  PSS : Inport  Port=4
  u : Inport  Port=5
  Complex to Magnitude-Angle : ComplexToMagnitudeAngle  Output=Magnitude
  Delta Pa PSS1 : spsGenericPowerSystemStabilizerLib/Generic Power System Stabilizer  Tsensor=15e-3  K=2.5*1.25  Twashout=1  Tleadlag1=[60e-3 1]  Tleadlag2=[0 0]  VSlimits=[-0.15 0.15]  Vinit=0  Plot_On=off  MagdB_On=on  FreqRange=logspace(-2,2,500)
  Delta w PSS (Kundur) : spsGenericPowerSystemStabilizerLib/Generic Power System Stabilizer  Tsensor=15e-3  K=30  Twashout=10  Tleadlag1=[50e-3 20e-3]  Tleadlag2=[3 5.4]  VSlimits=[-0.15 0.15]  Vinit=0  Plot_On=off  MagdB_On=on  FreqRange=logspace(-2,2,500)
  Demux : Demux  Outputs=2
      settings: DisplayOption=none
  Demux1 : Demux  Outputs=[2 1 1 1 1 1]
  EXCITATION : spsExcitationSystemLib/Excitation System  tr=20e-3  reg=[ 200, 0.001 ]  exc=[ 1, 0 ]  tgr=[ 0, 0 ]  damp=[ 0, 0 ]  sat=[ 0, 0 ]  lim=[ -12 , 12, 0 ]  v0=[1,1.83395]
  Goto3 : Goto  Commented=on  GotoTag=Pa2  TagVisibility=global
  Goto4 : Goto  Commented=on  GotoTag=pss2  TagVisibility=global
  Goto6 : Goto  Commented=on  GotoTag=Pe2  TagVisibility=global
  Goto7 : Goto  Commented=on  GotoTag=d_theta2  TagVisibility=global
  Multiport Switch : MultiPortSwitch  Inputs=4  SaturateOnIntegerOverflow=off
  PSS model1 : Constant  Value=0
  PSS model2 : Constant
  Real-Imag to Complex : RealImagToComplex
  STG : spsSteamTurbineandGovernorLib/Steam Turbine and Governor  gentype=Tandem-compound (single mass)  reg1="[ 1  0.05    0 ]"  reg2="[ 0.001  0.15 ]"  reg3="[ -0.1  0.1  0  4.496 ]"  N=3600  turb1="[ 0  10   3.3   0.5   ]"  turb2="[   0   0.36    0.36   0.28   ]"  HA="[ 0.046  1.430  1.465   0.192 ]"  KA="[ 90.44  53.88  64.59   62.94  ]"  DA="[ 0.0115  0.3575  0.3663   0.0137  ]"  ini1=0.7777  ini2=[0.779243,-42.8075]
  Sum1 : Sum  InputSameDT=on  SaturateOnIntegerOverflow=on  OutDataTypeStr=Inherit: Same as first input
  Sum2 : Sum  Inputs=-+  InputSameDT=on  SaturateOnIntegerOverflow=on  OutDataTypeStr=Inherit: Same as first input
  Sum3 : Sum  Inputs=|++
  Terminator{,1..3} (4 alike) : Terminator
  wref : Constant
  Pm : Outport  InitialOutput=0  VectorParamsAs1DForOutWhenUnconnected=off
  Vf : Outport  Port=2  InitialOutput=0  VectorParamsAs1DForOutWhenUnconnected=off
  tag scope: Vt2=global, w2=global
  wires:
  Sum2/1 -> Delta Pa PSS1/1, Goto3/1  "Pm-Pe"
  Demux1/5 -> Delta w PSS (Kundur)/1
  Demux1/4 -> Sum2/1, Goto6/1
  Demux1/3 -> [w2], STG/3
  Demux1/1 -> Demux/1
  PSS/1 -> Sum1/1
  Sum1/1 -> Multiport Switch/1
  PSS model2/1 -> Sum1/2
  Delta Pa PSS1/1 -> Multiport Switch/5
  Delta w PSS (Kundur)/1 -> Multiport Switch/4, Multiport Switch/3
  PSS model1/1 -> Multiport Switch/2
  Multiport Switch/1 -> Sum3/1, Goto4/1
  Demux1/6 -> Terminator3/1
  Complex to Magnitude-Angle/1 -> [Vt2]
  EXCITATION/1 -> Vf/1
  Real-Imag to Complex/1 -> Complex to Magnitude-Angle/1
  Vref/1 -> EXCITATION/1
  Pref/1 -> STG/2
  wref/1 -> STG/1
  Demux/2 -> Real-Imag to Complex/2, EXCITATION/3
  Demux/1 -> Real-Imag to Complex/1, EXCITATION/2
  STG/1 -> Terminator/1
  STG/2 -> Terminator1/1
  STG/3 -> Terminator2/1
  STG/4 -> Pm/1, Sum2/2
  Demux1/2 -> Goto7/1, STG/4
  m/1 -> Demux1/1
  u/1 -> Sum3/2
  Sum3/1 -> EXCITATION/4

== system Kundur_BESS_STA_Nov14_2021a_v2_2021a/Area 1/PI1 ==
  e(S) : Inport
  Add : Sum
  Integrator : Integrator  UpperSaturationLimit=1e2  LowerSaturationLimit=-1e2
  Ki : Gain  Gain=0.6
  Kp : Gain  Gain=0.3
  u(S) : Outport  VectorParamsAs1DForOutWhenUnconnected=off
  wires:
  Kp/1 -> Add/1
  e(S)/1 -> Ki/1, Kp/1
  Ki/1 -> Integrator/1
  Add/1 -> u(S)/1  "u(S)"
  Integrator/1 -> Add/2

== system Kundur_BESS_STA_Nov14_2021a_v2_2021a/Area 1/PI2 ==
  e(S) : Inport
  Add : Sum
  Integrator : Integrator  UpperSaturationLimit=1e2  LowerSaturationLimit=-1e2
  Ki : Gain  Gain=0.6
  Kp : Gain  Gain=0.3
  u(S) : Outport  VectorParamsAs1DForOutWhenUnconnected=off
  wires:
  Kp/1 -> Add/1
  e(S)/1 -> Ki/1, Kp/1
  Ki/1 -> Integrator/1
  Add/1 -> u(S)/1  "u(S)"
  Integrator/1 -> Add/2

== system Kundur_BESS_STA_Nov14_2021a_v2_2021a/Area 1/sig ==
  In1 : Inport
  Bus Selector1 : BusSelector  OutputSignals="dq0 components.Stator voltage  vq (pu),dq0 components.Stator voltage  vd (pu),Mechanical.Rotor angle deviation  d_theta (rad),Mechanical.Rotor speed  wm  (pu),Mechanical.Electrical power  Pe (pu),Mechanical.Rotor speed deviation  dw (pu),Mechanical.Rotor mechanical angle  theta (deg)"
  Mux : Mux  Inputs=6
  Mux1 : Mux  Inputs=2
  Out1 : Outport  VectorParamsAs1DForOutWhenUnconnected=off
  wires:
  Mux/1 -> Out1/1
  In1/1 -> Bus Selector1/1
  Bus Selector1/7 -> Mux/6  "<Rotor mechanical angle  theta (deg)>"
  Bus Selector1/6 -> Mux/5  "<Rotor speed deviation  dw (pu)>"
  Bus Selector1/5 -> Mux/4  "<Electrical power  Pe (pu)>"
  Bus Selector1/4 -> Mux/3  "<Rotor speed  wm  (pu)>"
  Bus Selector1/3 -> Mux/2  "<Rotor angle deviation  d_theta (rad)>"
  Bus Selector1/2 -> Mux1/2  "<Stator voltage  vd (pu)>"
  Bus Selector1/1 -> Mux1/1  "<Stator voltage  vq (pu)>"
  Mux1/1 -> Mux/1

== system Kundur_BESS_STA_Nov14_2021a_v2_2021a/Area 1/sig1 ==
  In1 : Inport
  Bus Selector1 : BusSelector  OutputSignals="dq0 components.Stator voltage  vq (pu),dq0 components.Stator voltage  vd (pu),Mechanical.Rotor angle deviation  d_theta (rad),Mechanical.Rotor speed  wm  (pu),Mechanical.Electrical power  Pe (pu),Mechanical.Rotor speed deviation  dw (pu),Mechanical.Rotor mechanical angle  theta (deg)"
  Mux : Mux  Inputs=6
  Mux1 : Mux  Inputs=2
  Out1 : Outport  VectorParamsAs1DForOutWhenUnconnected=off
  wires:
  Mux1/1 -> Mux/1
  Bus Selector1/1 -> Mux1/1  "<Stator voltage  vq (pu)>"
  Bus Selector1/2 -> Mux1/2  "<Stator voltage  vd (pu)>"
  Bus Selector1/3 -> Mux/2  "<Rotor angle deviation  d_theta (rad)>"
  Bus Selector1/4 -> Mux/3  "<Rotor speed  wm  (pu)>"
  Bus Selector1/5 -> Mux/4  "<Electrical power  Pe (pu)>"
  Bus Selector1/6 -> Mux/5  "<Rotor speed deviation  dw (pu)>"
  Bus Selector1/7 -> Mux/6  "<Rotor mechanical angle  theta (deg)>"
  In1/1 -> Bus Selector1/1
  Mux/1 -> Out1/1

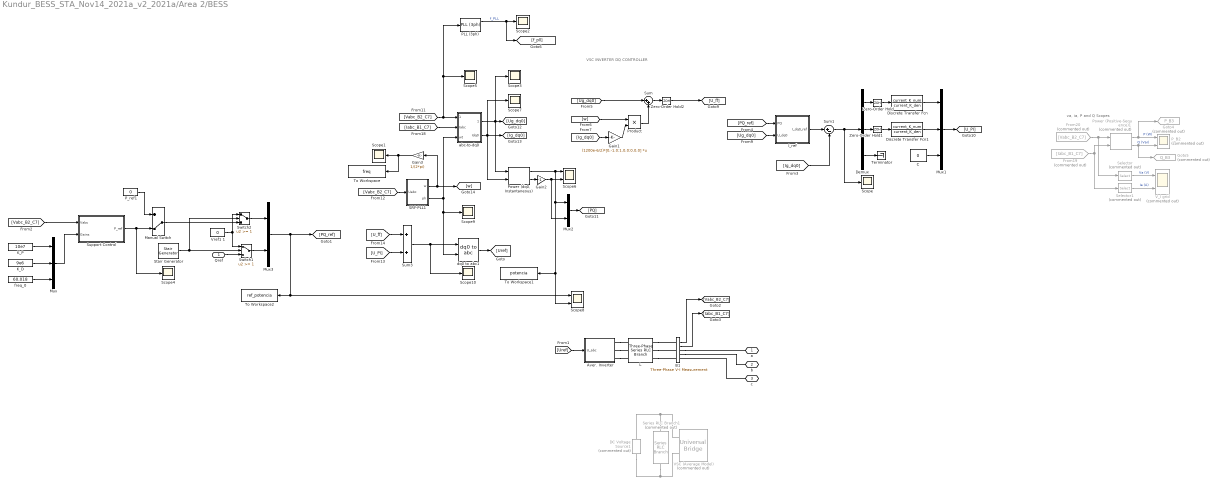
== system Kundur_BESS_STA_Nov14_2021a_v2_2021a/Area 2/BESS ==
  note: VSC INVERTER DQ CONTROLLER
  note: va, ia, P and Q Scopes
  Qref : Inport
  Aver. Inverter : Subsystem
  B1 : spsThreePhaseVIMeasurementLib/Three-Phase V-I Measurement  VoltageMeasurement=phase-to-ground  SetLabelV=off  LabelV=Vabc_B1  Vpu=off  VpuLL=off  CurrentMeasurement=yes  SetLabelI=off  LabelI=Iabc_B1_C7  Ipu=off  Pbase=100e6  Vbase=500e3  OutputType=Magnitude  PhasorSimulation=off  PSBequivalent=0
  C : Constant  Value=0
  DC Voltage Source1 : spsDCVoltageSourceLib/DC Voltage Source  Commented=on  Amplitude=Vdc  Measurements=None
  Demux : Demux  Outputs=3
  Discrete Transfer Fcn : DiscreteTransferFcn  Numerator=current_K_num  Denominator=current_K_den
  Discrete Transfer Fcn1 : DiscreteTransferFcn  Numerator=current_K_num  Denominator=current_K_den
  From19 : From  Commented=on  GotoTag=Iabc_B1_C7
      settings: CloseFcn=tagdialog Close
  From20 : From  Commented=on  GotoTag=Vabc_B2_C7
      settings: CloseFcn=tagdialog Close
  Gain1 : Gain  Gain=(1200e-6/2)*[0,-1,0;1,0,0;0,0,0]  Multiplication=Matrix(K*u)
  Gain2 : Gain  Gain=-1
  Gain3 : Gain  Gain=1/(2*pi)
  Goto4 : Goto  Commented=on  GotoTag=P_B3  TagVisibility=global
  Goto5 : Goto  Commented=on  GotoTag=Q_B3  TagVisibility=global
  I_ref : Subsystem
  K_D : Constant  Value=9e6
  K_P : Constant  Value=10e7
  L : spsThreePhaseSeriesRLCBranchLib/Three-Phase Series RLC Branch  LConnTagsString=A|B|C  RConnTagsString=A|B|C  BranchType=RL  Resistance=500e-6*377/50/2  Inductance=1200e-6/2  Capacitance=inf  Measurements=None
  Manual Switch : ManualSwitch  CurrentSetting=0
  Mux : Mux  Inputs=3
  Mux1 : Mux  Inputs=3
  Mux2 : Mux  Inputs=2
  Mux3 : Mux  Inputs=2
  PLL (3ph) : spsPLL3phLib/PLL (3ph)  Fmin=58  Par_Init="[-0.57  60]"  ParK=[180, 3200, 0.1]  TcD=1e-4  MaxRateChangeFreq=5  FilterCutOffFreq=5  Ts=Ts  AGC=on
  P_B2 : Scope  Commented=on  NumInputPorts=2
  P_ref1 : Constant  Value=0
  Power (Positive-Sequence)1 : spsPowerPositiveSequenceLib/Power (Positive-Sequence)  Commented=on  Freq=60  Vinit=[0, 0]  Iinit=[0, 0]  Ts=Ts
  "Power (dq0, Instantaneous)" : spsPowerdq0InstantaneousLib/Power (dq0, Instantaneous)
  Product : Product
  SRF-PLL1 : Subsystem
  Scope{,1..5,7,9..10} (9 alike) : Scope
  Scope6 : Scope  NumInputPorts=2
  Scope8 : Scope  NumInputPorts=2
  Selector : Selector  Commented=on  InputPortWidth=3  IndexOptions=Index vector (dialog)  Indices=[1]  OutputSizes=1
  Selector1 : Selector  Commented=on  InputPortWidth=3  IndexOptions=Index vector (dialog)  Indices=[1]  OutputSizes=1
  Series RLC Branch1 : spsSeriesRLCBranchLib/Series RLC Branch  Commented=on  LConnTagsString=__new0  RConnTagsString=__new0  BranchType=RC  Resistance=1e-7  Inductance=1e-3  SetiL0=off  InitialCurrent=0  Capacitance=C  Setx0=off  InitialVoltage=400  Measurements=None
  Stair Generator : spsStairGeneratorLib/Stair Generator  t=[0 1]  e=[1 0]  Ts=0
  Sum : Sum  Inputs=|++
  Sum1 : Sum  Inputs=|+-
  Sum3 : Sum
  Support Control : Subsystem  Variant=on
  Switch1 : Switch  Threshold=1  SaturateOnIntegerOverflow=off
  Switch2 : Switch  Threshold=1  SaturateOnIntegerOverflow=off
  Terminator : Terminator
  To Workspace : ToWorkspace  VariableName=freq  SaveFormat=Timeseries  SampleTime=1e-4
  To Workspace1 : ToWorkspace  VariableName=potencia  SaveFormat=Timeseries  SampleTime=1e-4
  To Workspace2 : ToWorkspace  VariableName=ref_potencia  SaveFormat=Timeseries  SampleTime=1e-4
  VSC (Average Model) : spsUniversalBridgeLib/Universal Bridge  Commented=on  Arms=3  SnubberResistance=1e5  SnubberCapacitance=inf  Device=Average-model based VSC  Ron=1e-3  Lon=0  ForwardVoltages="[  0  0  ]"  ForwardVoltage=0  GTOparameters=[ 10e-6 , 20e-6 ]  IGBTparameters=[ 1e-6 , 2e-6 ]  Measurements=None  Measurements_2=None  converterType=Rectifier
  V_I grid : Scope  Commented=on  NumInputPorts=2
  Vref1 1 : Constant  Value=0
  Zero-Order Hold : ZeroOrderHold  SampleTime=sampling_k
  Zero-Order Hold1 : ZeroOrderHold  SampleTime=sampling_k
  Zero-Order Hold2 : ZeroOrderHold  SampleTime=sampling_k
  abc-to-dq0 : Subsystem
  dq0 to abc1 : spsdq0toabcLib/dq0 to abc  Alignment=90 degrees behind phase A axis
  freq_0 : Constant  Value=60.018
  a : PMIOPort  Side=Right
  b : PMIOPort  Port=2  Side=Right
  c : PMIOPort  Port=3  Side=Right
  wires:
  Selector/1 -> V_I grid/1  "Va (V)"
  Power (Positive-Sequence)1/2 -> Goto5/1, P_B2/2  "Q (Var)"
  From20/1 -> Selector/1, Power (Positive-Sequence)1/1
  Selector1/1 -> V_I grid/2  "Ia (A)"
  From19/1 -> Power (Positive-Sequence)1/2, Selector1/1
  Power (Positive-Sequence)1/1 -> Goto4/1, P_B2/1  "P (W)"
  B1/1 -> [Vabc_B2_C7]
  B1/2 -> [Iabc_B1_C7]
  freq_0/1 -> Mux/3
  P_ref1/1 -> Manual Switch/1
  [Vabc_B2_C7] -> Support Control/1(Vabc)
  K_D/1 -> Mux/2
  Mux/1 -> Support Control/2(Gains)
  Support Control/1(P_ref) -> Scope4/1, Manual Switch/2
  K_P/1 -> Mux/1
  Qref/1 -> Switch1/3
  Stair Generator/1 -> Switch2/2, Switch1/2
  Vref1 1/1 -> Switch2/1, Switch1/1
  Manual Switch/1 -> Switch2/3
  [Ug_dq0] -> Sum/1
  Gain1/1 -> Product/2
  [w] -> Product/1
  Product/1 -> Sum/2
  [Vabc_B2_C7] -> PLL (3ph)/1, Scope5/1, abc-to-dq0/1(Uabc)
  [Vabc_B2_C7] -> SRF-PLL1/1(Uabc)
  Gain3/1 -> To Workspace/1, Scope1/1
  SRF-PLL1/1(w) -> Gain3/1, [w]
  "Power (dq0, Instantaneous)"/1 -> Scope6/1, Mux2/1, To Workspace1/1, Scope8/2
  Mux2/1 -> [PQ]
  [U_ff] -> Sum3/1
  SRF-PLL1/2(ph) -> Scope9/1, dq0 to abc1/2, abc-to-dq0/3(wt)
  [U_PI] -> Sum3/2
  Switch2/1 -> Mux3/1
  Switch1/1 -> Mux3/2
  Mux3/1 -> To Workspace2/1, Scope8/1, [PQ_ref]
  [Ug_dq0] -> I_ref/2(U_dq0)
  [PQ_ref] -> I_ref/1(PQ)
  Demux/3 -> Terminator/1
  C/1 -> Mux1/3
  [Ig_dq0] -> Sum1/2
  Sum1/1 -> Demux/1, Scope/1
  Demux/1 -> Zero-Order Hold/1
  Demux/2 -> Zero-Order Hold1/1
  I_ref/1(I_dq0_ref) -> Sum1/1
  Mux1/1 -> [U_PI]
  [Iabc_B1_C7] -> abc-to-dq0/2(Iabc)
  abc-to-dq0/2(Idq0) -> "Power (dq0, Instantaneous)"/2, Scope7/1, [Ig_dq0]
  abc-to-dq0/1(Udq0) -> Scope3/1, [Ug_dq0], "Power (dq0, Instantaneous)"/1
  "Power (dq0, Instantaneous)"/2 -> Gain2/1
  Gain2/1 -> Mux2/2, Scope6/2
  [Ig_dq0] -> Gain1/1
  Zero-Order Hold/1 -> Discrete Transfer Fcn/1
  Zero-Order Hold1/1 -> Discrete Transfer Fcn1/1
  Discrete Transfer Fcn/1 -> Mux1/1
  Discrete Transfer Fcn1/1 -> Mux1/2
  Sum/1 -> Zero-Order Hold2/1
  [Uref] -> Aver. Inverter/1(U_abc)
  PLL (3ph)/1 -> [f_pll], Scope2/1  "f_PLL"
  Sum3/1 -> Scope10/1, dq0 to abc1/1
  dq0 to abc1/1 -> [Uref]
  Zero-Order Hold2/1 -> [U_ff]
  connections:
  Series RLC Branch1/RConn1 -- DC Voltage Source1/LConn1 -- VSC (Average Model)/RConn2
  c/RConn1 -- B1/RConn3
  DC Voltage Source1/RConn1 -- VSC (Average Model)/RConn1 -- Series RLC Branch1/LConn1
  B1/RConn1 -- a/RConn1
  B1/RConn2 -- b/RConn1
  Aver. Inverter/RConn2 -- L/LConn2
  Aver. Inverter/RConn1 -- L/LConn1
  Aver. Inverter/RConn3 -- L/LConn3
  L/RConn1 -- B1/LConn1
  L/RConn2 -- B1/LConn2
  L/RConn3 -- B1/LConn3

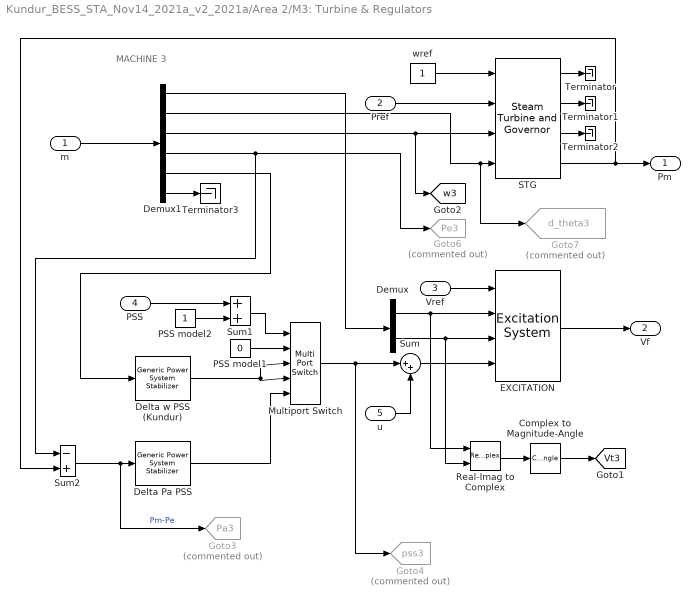
== system Kundur_BESS_STA_Nov14_2021a_v2_2021a/Area 2/M3: Turbine & Regulators ==
  note: MACHINE 3
  m : Inport
  Pref : Inport  Port=2
  Vref : Inport  Port=3
  PSS : Inport  Port=4
  u : Inport  Port=5
  Complex to Magnitude-Angle : ComplexToMagnitudeAngle  Output=Magnitude
  Delta Pa PSS : spsGenericPowerSystemStabilizerLib/Generic Power System Stabilizer  Tsensor=15e-3  K=2.5*1.25  Twashout=1  Tleadlag1=[60e-3 1]  Tleadlag2=[0 0]  VSlimits=[-0.15 0.15]  Vinit=0  Plot_On=off  MagdB_On=on  FreqRange=logspace(-2,2,500)
  Delta w PSS (Kundur) : spsGenericPowerSystemStabilizerLib/Generic Power System Stabilizer  Tsensor=15e-3  K=30  Twashout=10  Tleadlag1=[50e-3 20e-3]  Tleadlag2=[3 5.4]  VSlimits=[-0.15 0.15]  Vinit=0  Plot_On=off  MagdB_On=on  FreqRange=logspace(-2,2,500)
  Demux : Demux  Outputs=2
      settings: DisplayOption=none
  Demux1 : Demux  Outputs=[2 1 1 1 1 1]
  EXCITATION : spsExcitationSystemLib/Excitation System  tr=20e-3  reg=[ 200, 0.001 ]  exc=[ 1, 0 ]  tgr=[ 0, 0 ]  damp=[ 0, 0 ]  sat=[ 0, 0 ]  lim=[ -12.3 , 12.3, 0 ]  v0=[1,1.83395]
  Goto3 : Goto  Commented=on  GotoTag=Pa3  TagVisibility=global
  Goto4 : Goto  Commented=on  GotoTag=pss3  TagVisibility=global
  Goto6 : Goto  Commented=on  GotoTag=Pe3  TagVisibility=global
  Goto7 : Goto  Commented=on  GotoTag=d_theta3  TagVisibility=global
  Multiport Switch : MultiPortSwitch  Inputs=4  SaturateOnIntegerOverflow=off
  PSS model1 : Constant  Value=0
  PSS model2 : Constant
  Real-Imag to Complex : RealImagToComplex
  STG : spsSteamTurbineandGovernorLib/Steam Turbine and Governor  gentype=Tandem-compound (single mass)  reg1="[ 1  0.05    0 ]"  reg2="[ 0.001  0.15 ]"  reg3="[ -0.1  0.1  0  4.496 ]"  N=3600  turb1="[ 0  10   3.3   0.5   ]"  turb2="[   0   0.36    0.36   0.28   ]"  HA="[ 0.046  1.430  1.465   0.192 ]"  KA="[ 90.44  53.88  64.59   62.94  ]"  DA="[ 0.0115  0.3575  0.3663   0.0137  ]"  ini1=0.798889  ini2=[0.800505,-56.3243]
  Sum : Sum  Inputs=|++
  Sum1 : Sum  InputSameDT=on  SaturateOnIntegerOverflow=on  OutDataTypeStr=Inherit: Same as first input
  Sum2 : Sum  Inputs=-+  InputSameDT=on  SaturateOnIntegerOverflow=on  OutDataTypeStr=Inherit: Same as first input
  Terminator{,1..3} (4 alike) : Terminator
  wref : Constant
  Pm : Outport  InitialOutput=0  VectorParamsAs1DForOutWhenUnconnected=off
  Vf : Outport  Port=2  InitialOutput=0  VectorParamsAs1DForOutWhenUnconnected=off
  tag scope: Vt3=global, w3=global
  wires:
  Sum2/1 -> Goto3/1, Delta Pa PSS/1  "Pm-Pe"
  Demux1/5 -> Delta w PSS (Kundur)/1
  Demux1/4 -> Sum2/1, Goto6/1
  Demux1/3 -> [w3], STG/3
  Demux1/1 -> Demux/1
  PSS/1 -> Sum1/1
  Sum1/1 -> Multiport Switch/1
  PSS model2/1 -> Sum1/2
  Delta Pa PSS/1 -> Multiport Switch/5
  Delta w PSS (Kundur)/1 -> Multiport Switch/4, Multiport Switch/3
  PSS model1/1 -> Multiport Switch/2
  Multiport Switch/1 -> Goto4/1, Sum/1
  Demux1/6 -> Terminator3/1
  Complex to Magnitude-Angle/1 -> [Vt3]
  EXCITATION/1 -> Vf/1
  Real-Imag to Complex/1 -> Complex to Magnitude-Angle/1
  Vref/1 -> EXCITATION/1
  m/1 -> Demux1/1
  Pref/1 -> STG/2
  wref/1 -> STG/1
  Demux/2 -> Real-Imag to Complex/2, EXCITATION/3
  Demux/1 -> Real-Imag to Complex/1, EXCITATION/2
  Demux1/2 -> Goto7/1, STG/4
  STG/1 -> Terminator/1
  STG/2 -> Terminator1/1
  STG/3 -> Terminator2/1
  STG/4 -> Pm/1, Sum2/2
  u/1 -> Sum/2
  Sum/1 -> EXCITATION/4

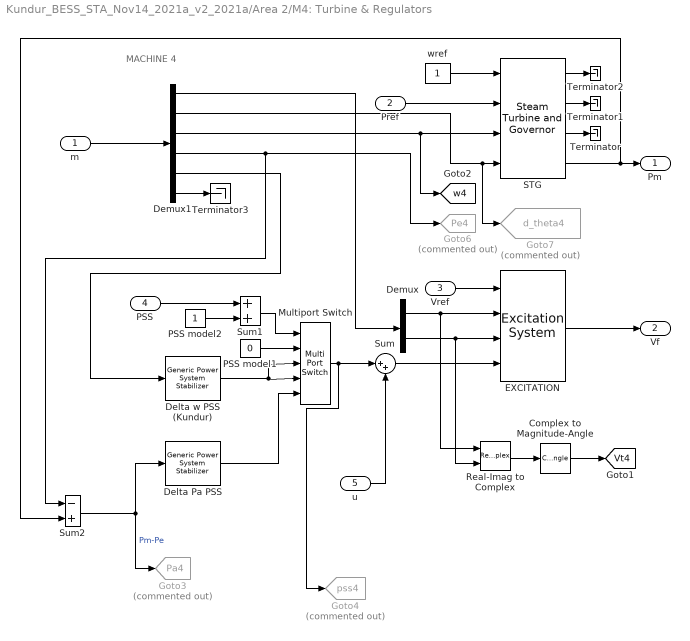
== system Kundur_BESS_STA_Nov14_2021a_v2_2021a/Area 2/M4: Turbine & Regulators ==
  note: MACHINE 4
  m : Inport
  Pref : Inport  Port=2
  Vref : Inport  Port=3
  PSS : Inport  Port=4
  u : Inport  Port=5
  Complex to Magnitude-Angle : ComplexToMagnitudeAngle  Output=Magnitude
  "Delta Pa PSS " : spsGenericPowerSystemStabilizerLib/Generic Power System Stabilizer  Tsensor=15e-3  K=2.5*1.25  Twashout=1  Tleadlag1=[60e-3 1]  Tleadlag2=[0 0]  VSlimits=[-0.15 0.15]  Vinit=0  Plot_On=off  MagdB_On=on  FreqRange=logspace(-2,2,500)
  Delta w PSS (Kundur) : spsGenericPowerSystemStabilizerLib/Generic Power System Stabilizer  Tsensor=15e-3  K=30  Twashout=10  Tleadlag1=[50e-3 20e-3]  Tleadlag2=[3 5.4]  VSlimits=[-0.15 0.15]  Vinit=0  Plot_On=off  MagdB_On=on  FreqRange=logspace(-2,2,500)
  Demux : Demux  Outputs=2
      settings: DisplayOption=none
  Demux1 : Demux  Outputs=[2 1 1 1 1 1]
  EXCITATION : spsExcitationSystemLib/Excitation System  tr=20e-3  reg=[ 200, 0.001 ]  exc=[ 1, 0 ]  tgr=[ 0, 0 ]  damp=[ 0, 0 ]  sat=[ 0, 0 ]  lim=[ -12.3 , 12.3, 0 ]  v0=[1,1.83395]
  Goto3 : Goto  Commented=on  GotoTag=Pa4  TagVisibility=global
  Goto4 : Goto  Commented=on  GotoTag=pss4  TagVisibility=global
  Goto6 : Goto  Commented=on  GotoTag=Pe4  TagVisibility=global
  Goto7 : Goto  Commented=on  GotoTag=d_theta4  TagVisibility=global
  Multiport Switch : MultiPortSwitch  Inputs=4  SaturateOnIntegerOverflow=off
  PSS model1 : Constant  Value=0
  PSS model2 : Constant
  Real-Imag to Complex : RealImagToComplex
  STG : spsSteamTurbineandGovernorLib/Steam Turbine and Governor  gentype=Tandem-compound (single mass)  reg1="[ 1  0.05    0 ]"  reg2="[ 0.001  0.15 ]"  reg3="[ -0.1  0.1  0  4.496 ]"  N=3600  turb1="[ 0  10   3.3   0.5   ]"  turb2="[   0   0.36    0.36   0.28   ]"  HA="[ 0.046  1.430  1.465   0.192 ]"  KA="[ 90.44  53.88  64.59   62.94  ]"  DA="[ 0.0115  0.3575  0.3663   0.0137  ]"  ini1=0.7778  ini2=[0.779311,-67.7513]
  Sum : Sum  Inputs=|++
  Sum1 : Sum  InputSameDT=on  SaturateOnIntegerOverflow=on  OutDataTypeStr=Inherit: Same as first input
  Sum2 : Sum  Inputs=-+  InputSameDT=on  SaturateOnIntegerOverflow=on  OutDataTypeStr=Inherit: Same as first input
  Terminator{,1..3} (4 alike) : Terminator
  wref : Constant
  Pm : Outport  InitialOutput=0  VectorParamsAs1DForOutWhenUnconnected=off
  Vf : Outport  Port=2  InitialOutput=0  VectorParamsAs1DForOutWhenUnconnected=off
  tag scope: Vt4=global, w4=global
  wires:
  Demux/1 -> Real-Imag to Complex/1, EXCITATION/2
  Demux/2 -> Real-Imag to Complex/2, EXCITATION/3
  STG/4 -> Pm/1, Sum2/2
  wref/1 -> STG/1
  Pref/1 -> STG/2
  m/1 -> Demux1/1
  Vref/1 -> EXCITATION/1
  STG/3 -> Terminator/1
  Real-Imag to Complex/1 -> Complex to Magnitude-Angle/1
  EXCITATION/1 -> Vf/1
  Complex to Magnitude-Angle/1 -> [Vt4]
  Demux1/6 -> Terminator3/1
  Multiport Switch/1 -> Sum/1, Goto4/1
  PSS model1/1 -> Multiport Switch/2
  Delta w PSS (Kundur)/1 -> Multiport Switch/4, Multiport Switch/3
  "Delta Pa PSS "/1 -> Multiport Switch/5
  PSS model2/1 -> Sum1/2
  Sum1/1 -> Multiport Switch/1
  PSS/1 -> Sum1/1
  Demux1/1 -> Demux/1
  Demux1/3 -> [w4], STG/3
  Demux1/4 -> Sum2/1, Goto6/1
  Demux1/5 -> Delta w PSS (Kundur)/1
  Sum2/1 -> "Delta Pa PSS "/1, Goto3/1  "Pm-Pe"
  STG/2 -> Terminator1/1
  STG/1 -> Terminator2/1
  Demux1/2 -> Goto7/1, STG/4
  u/1 -> Sum/2
  Sum/1 -> EXCITATION/4

== system Kundur_BESS_STA_Nov14_2021a_v2_2021a/Area 2/PI1 ==
  e(S) : Inport
  Add : Sum
  Integrator : Integrator  UpperSaturationLimit=1e2  LowerSaturationLimit=-1e2
  Ki : Gain  Gain=0.6
  Kp : Gain  Gain=0.3
  u(S) : Outport  VectorParamsAs1DForOutWhenUnconnected=off
  wires:
  Kp/1 -> Add/1
  e(S)/1 -> Ki/1, Kp/1
  Ki/1 -> Integrator/1
  Add/1 -> u(S)/1  "u(S)"
  Integrator/1 -> Add/2

== system Kundur_BESS_STA_Nov14_2021a_v2_2021a/Area 2/PI3 ==
  e(S) : Inport
  Add : Sum
  Integrator : Integrator  UpperSaturationLimit=1e2  LowerSaturationLimit=-1e2
  Ki : Gain  Gain=0.6
  Kp : Gain  Gain=0.3
  u(S) : Outport  VectorParamsAs1DForOutWhenUnconnected=off
  wires:
  Kp/1 -> Add/1
  e(S)/1 -> Ki/1, Kp/1
  Ki/1 -> Integrator/1
  Add/1 -> u(S)/1  "u(S)"
  Integrator/1 -> Add/2
